simulink model "imsimulation"  (R2013a)
settings: Solver=ode45  StartTime=0.0  StopTime=10  RelTol=1e-3
values from neighbouring files (symbols this model uses):
  J = 0.089    [matlab.mat]
  P = 4    [matlab.mat]
  Rr = 0.816    [matlab.mat]
  Rs = 0.49    [matlab.mat]
  theta = 0    [matlab.mat]
  Wb = 157    [matlab.mat]
  We = 157    [matlab.mat]
  Xlr = 0.754    [matlab.mat]
  Xls = 0.754    [matlab.mat]
  Xm = 26.13    [matlab.mat]
undefined symbols (not defined in the file or in its folder): sigbuilder_block
settings Model: Creator=Administrator  LastModifiedBy=User
settings DebuggingCC: MultiTaskDSMMsg=warning  MultiTaskCondExecSysMsg=none  FcnCallInpInsideContextMsg=EnableAllAsWarning  StrictBusMsg=None
settings RTWCC: IncludeERTFirstTime=on

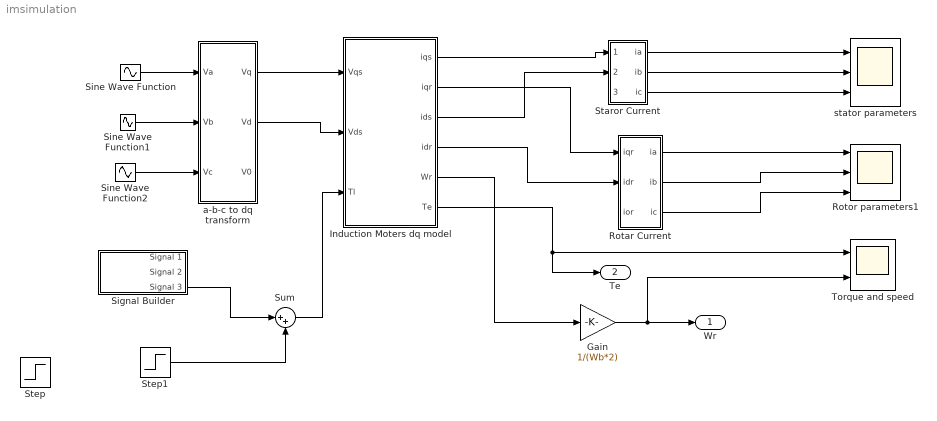
== system imsimulation ==
  Gain : Gain  Gain=1/(Wb*2)
  "Induction Moters dq model " : Subsystem
  Rotar Current : Subsystem
  Rotor parameters1 : Scope  NumInputPorts=3
      settings: YMin=-5~-5~-5  YMax=5~5~5
  Signal Builder : Subsystem  Tag=STV Subsys  LoadFcn=sigbuilder_block('load');  StartFcn=sigbuilder_block('start');  StopFcn=sigbuilder_block('stop');  ClipboardFcn=sigbuilder_block('clipboard');  mask(Sigbuilder block){}
      mask help: Simulink:masks:SigbuilderBlock_MD
      mask init:
      | if ~strcmp(get_param(bdroot(gcbh),'SimulationStatus'),'stopped') tuvar = sigbuilder_block('maskInit'); end
      settings: CopyFcn=sigbuilder_block('copy');  DeleteFcn=sigbuilder_block('delete');  ModelCloseFcn=sigbuilder_block('modelClose');  PreSaveFcn=sigbuilder_block('preSave');  PauseFcn=sigbuilder_block('pause');  ContinueFcn=sigbuilder_block('continue');  NameChangeFcn=sigbuilder_block('namechange');  OpenFcn=sigbuilder_block('open',[6 30.75 1012.5 481.5 ]);  CloseFcn=sigbuilder_block('close');
      mask Display: plot(0, 0, 100, 100,[2, 2, 32, 32, 2], [68, 8, 8, 68, 68],[32, 2], [38, 38], [32, 19, 2],[53, 60, 44], [32, 17, 17, 2],[16, 16, 31, 31]);txt = getActiveGroup(gcbh);text(2, 100, txt,'verticalAlignment', 'top');
  Sine Wave Function : Sin  Amplitude=311.11  Frequency=50*2*pi  SampleTime=0
  Sine Wave Function1 : Sin  Amplitude=311.11  Frequency=50*2*pi  Phase=0-(2*pi/3)  SampleTime=0
  Sine Wave Function2 : Sin  Amplitude=311.11  Frequency=50*2*pi  Phase=0+(2*pi/3)  SampleTime=0
  "Staror Current " : Subsystem
  Step : Step  Time=3  After=11.95  SampleTime=0
  Step1 : Step  Time=6  After=-11.9  SampleTime=0
  Sum : Sum  Inputs=|++
  "Torque and speed " : Scope  NumInputPorts=2
      settings: TimeRange=0.1239454679989271  YMin=-60~-0.2  YMax=100~1.6  SaveName=ScopeData2
  "a-b-c to dq transform " : Subsystem
  stator parameters : Scope  NumInputPorts=3
      settings: TimeRange=1  YMin=-100~-100~-100  YMax=100~100~100
  Wr : Outport
  Te : Outport  Port=2
  wires:
  Sine Wave Function/1 -> "a-b-c to dq transform "/1(Va)
  Sine Wave Function1/1 -> "a-b-c to dq transform "/2(Vb)
  Sine Wave Function2/1 -> "a-b-c to dq transform "/3(Vc)
  "a-b-c to dq transform "/1(Vq) -> "Induction Moters dq model "/1(Vqs)
  "a-b-c to dq transform "/2(Vd) -> "Induction Moters dq model "/2(Vds)
  "Induction Moters dq model "/1(iqs) -> "Staror Current "/1(iqs)
  "Induction Moters dq model "/3(ids) -> "Staror Current "/2(ids)
  "Induction Moters dq model "/4(idr) -> Rotar Current/2(idr)
  "Induction Moters dq model "/2(iqr) -> Rotar Current/1(iqr)
  "Staror Current "/1(ia) -> stator parameters/1
  Rotar Current/1(ia) -> Rotor parameters1/1
  Rotar Current/2(ib) -> Rotor parameters1/2
  "Induction Moters dq model "/6(Te) -> Te/1, "Torque and speed "/1
  Step1/1 -> Sum/2
  "Induction Moters dq model "/5(Wr) -> Gain/1
  Sum/1 -> "Induction Moters dq model "/3(Tl)
  Gain/1 -> "Torque and speed "/2, Wr/1
  "Staror Current "/2(ib) -> stator parameters/2
  "Staror Current "/3("ic ") -> stator parameters/3
  Rotar Current/3("ic ") -> Rotor parameters1/3
  Signal Builder/3(Signal 3) -> Sum/1

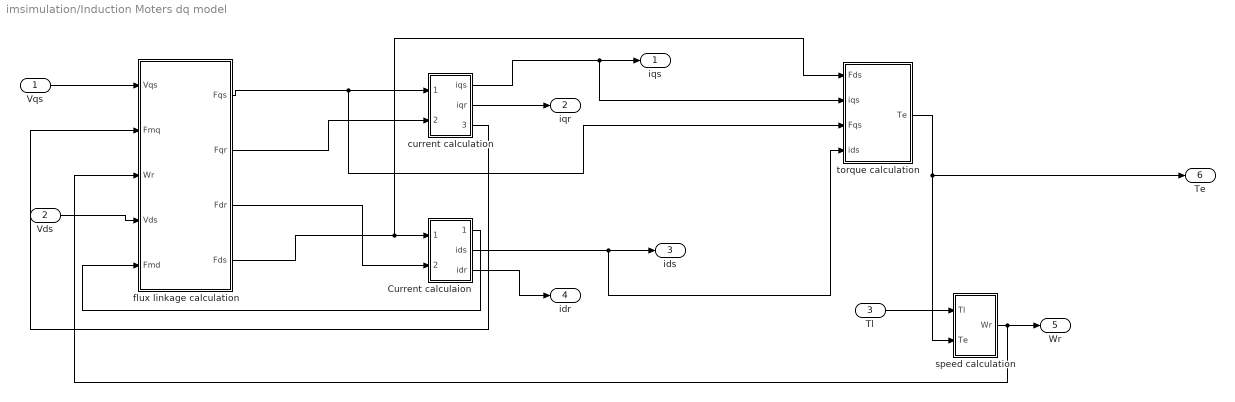
== system imsimulation/Induction Moters dq model  ==
  Vqs : Inport
  Vds : Inport  Port=2
  Tl : Inport  Port=3
  "Current calculaion " : Subsystem
  current calculation : Subsystem
  flux linkage calculation : Subsystem
  speed calculation : Subsystem
  "torque calculation " : Subsystem
  iqs : Outport
  iqr : Outport  Port=2
  ids : Outport  Port=3
  idr : Outport  Port=4
  Wr : Outport  Port=5
  Te : Outport  Port=6
  wires:
  Tl/1 -> speed calculation/1(Tl)
  "Current calculaion "/1(Fmd) -> flux linkage calculation/5(Fmd)
  current calculation/2(iqr) -> iqr/1
  current calculation/1(iqs) -> iqs/1, "torque calculation "/2(iqs)
  flux linkage calculation/3(Fdr) -> "Current calculaion "/2(Fdr)
  "Current calculaion "/2(ids) -> ids/1, "torque calculation "/4(ids)
  "Current calculaion "/3(idr) -> idr/1
  "torque calculation "/1(Te) -> Te/1, speed calculation/2(Te)
  flux linkage calculation/1(Fqs) -> "torque calculation "/3(Fqs), current calculation/1(Fqs)
  Vqs/1 -> flux linkage calculation/1(Vqs)
  Vds/1 -> flux linkage calculation/4(Vds)
  flux linkage calculation/2(Fqr) -> current calculation/2(Fqr)
  current calculation/3(Fmq) -> flux linkage calculation/2(Fmq)
  speed calculation/1(Wr) -> Wr/1, flux linkage calculation/3(Wr)
  flux linkage calculation/4(Fds) -> "torque calculation "/1(Fds), "Current calculaion "/1(Fds)

== system imsimulation/Rotar Current ==
  iqr : Inport
  idr : Inport  Port=2
  ior : Inport  Port=3
  Subsystem : Subsystem
  Subsystem1 : Subsystem
  Subsystem2 : Subsystem
  ia : Outport
  ib : Outport  Port=2
  "ic " : Outport  Port=3
  wires:
  Subsystem2/1("ic ") -> "ic "/1
  Subsystem1/1(ib) -> ib/1
  ior/1 -> Subsystem2/3(i0r), Subsystem/3(i0r), Subsystem1/3(i0r)
  idr/1 -> Subsystem2/2(idr), Subsystem/2(idr), Subsystem1/2(idr)
  iqr/1 -> Subsystem/1(iqr), Subsystem1/1(iqr), Subsystem2/1(iqr)
  Subsystem/1(ia) -> ia/1

== system imsimulation/Signal Builder ==
  Demux : Demux  Tag=STV Demux  Outputs=3
  FromWs : FromWorkspace  Tag=STV FromWs  VariableName=tuvar  SampleTime=0
      SigBuilderData=|
      | common.afterFinalStr = 'Extrapolate'
      | common.sampleTime = 0
      | dataSet.timeRange = [0 10]
      | dataSet.name = 'Group 1'
      | sbobj.Groups.Name = 'Group 1'
      | sbobj.Groups.Signals(1).Name = 'Signal 1'
      | sbobj.Groups.Signals(1).XData = [0 4 6 6 10]
      | sbobj.Groups.Signals(1).YData = [0 1.005 1 1.005 0.995]
      | sbobj.Groups.Signals(2).Name = 'Signal 2'
      | sbobj.Groups.Signals(2).XData = [0 0.5 0.5 1 1 1.5 1.5 2 2 2.5 2.5 3 3 3.5 3.5 4 4 4.5 4.5 5 5 5.5 5.5 6 6 6.5 6.5 7 7 7.5 7.5 8 8 8.5 8.5 9 9 9.5 9.5 10]
      | sbobj.Groups.Signals(2).YData = [2 2 0 0 2 2 0 0 2 2 0 0 2 2 0 0 2 2 0 0 2 2 0 0 2 2 0 0 2 2 0 0 2 2 0 0 2 2 0 0]
      | sbobj.Groups.Signals(3).Name = 'Signal 3'
      | sbobj.Groups.Signals(3).XData = [0 10]
      | sbobj.Groups.Signals(3).YData = [1 1]
  Signal 1 : Outport  Tag=STV Outport
  Signal 2 : Outport  Tag=STV Outport  Port=2
  Signal 3 : Outport  Tag=STV Outport  Port=3
  wires:
  Demux/1 -> Signal 1/1
  FromWs/1 -> Demux/1
  Demux/2 -> Signal 2/1
  Demux/3 -> Signal 3/1

== system imsimulation/Staror Current  ==
  iqs : Inport
  ids : Inport  Port=2
  ios : Inport  Port=3
  Subsystem : Subsystem
  Subsystem1 : Subsystem
  Subsystem2 : Subsystem
  ia : Outport
  ib : Outport  Port=2
  "ic " : Outport  Port=3
  wires:
  Subsystem/1(ia) -> ia/1
  iqs/1 -> Subsystem2/1(iqs), Subsystem1/1(iqs), Subsystem/1(iqs)
  ids/1 -> Subsystem1/2(ids), Subsystem/2(ids), Subsystem2/2(ids)
  ios/1 -> Subsystem1/3(i0s), Subsystem/3(i0s), Subsystem2/3(i0)
  Subsystem1/1(ib) -> ib/1
  Subsystem2/1("ic ") -> "ic "/1

== system imsimulation/a-b-c to dq transform  ==
  Va : Inport
  Vb : Inport  Port=2
  Vc : Inport  Port=3
  Subsystem : Subsystem
  Subsystem1 : Subsystem
  Subsystem2 : Subsystem
  Vq : Outport
  Vd : Outport  Port=2
  V0 : Outport  Port=3
  wires:
  Vc/1 -> Subsystem2/3(Vc), Subsystem1/3(Vc), Subsystem/3(Vc)
  Vb/1 -> Subsystem/2(Vb), Subsystem1/2(Vb), Subsystem2/2(Vb)
  Subsystem/1(Vq) -> Vq/1
  Subsystem1/1("Vd ") -> Vd/1
  Va/1 -> Subsystem1/1(Va), Subsystem/1(Va), Subsystem2/1(Va)
  Subsystem2/1(V0) -> V0/1

== system imsimulation/Induction Moters dq model /Current calculaion  ==
  Fds : Inport
  Fdr : Inport  Port=2
  Subsystem1 : Subsystem
  Subsystem4 : Subsystem
  Subsystem5 : Subsystem
  Fmd : Outport
  ids : Outport  Port=2
  idr : Outport  Port=3
  wires:
  Subsystem1/1(Fmd) -> Fmd/1, Subsystem4/2(Fmd), Subsystem5/2(Fmd)
  Fdr/1 -> Subsystem5/1(Fdr), Subsystem1/2(Fdr)
  Fds/1 -> Subsystem4/1(Fds), Subsystem1/1(Fds)
  Subsystem4/1(ids) -> ids/1
  Subsystem5/1(idr) -> idr/1

== system imsimulation/Induction Moters dq model /current calculation ==
  Fqs : Inport
  Fqr : Inport  Port=2
  Subsystem : Subsystem
  Subsystem2 : Subsystem
  Subsystem3 : Subsystem
  iqs : Outport
  iqr : Outport  Port=2
  Fmq : Outport  Port=3
  wires:
  Subsystem2/1(iqs) -> iqs/1
  Subsystem/1(Fmq) -> Fmq/1, Subsystem2/2(Fmq), Subsystem3/2(Fmq)
  Subsystem3/1(iqr) -> iqr/1
  Fqs/1 -> Subsystem/1(Fqs), Subsystem2/1(Fqs)
  Fqr/1 -> Subsystem/2(Fqr), Subsystem3/1(Fqr)

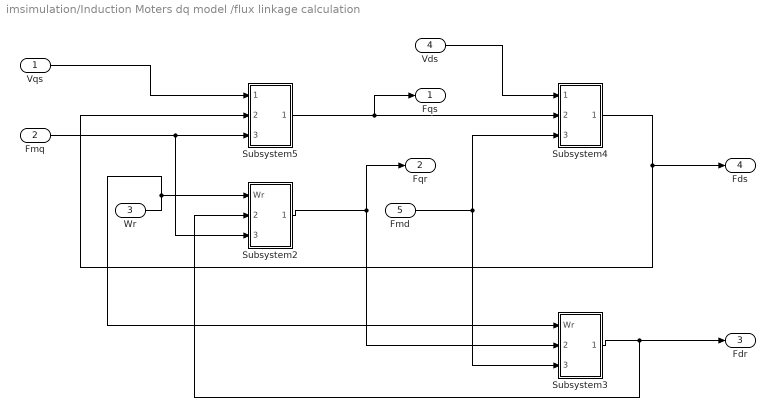
== system imsimulation/Induction Moters dq model /flux linkage calculation ==
  Vqs : Inport
  Fmq : Inport  Port=2
  Wr : Inport  Port=3
  Vds : Inport  Port=4
  Fmd : Inport  Port=5
  Subsystem2 : Subsystem
  Subsystem3 : Subsystem
  Subsystem4 : Subsystem
  Subsystem5 : Subsystem
  Fqs : Outport
  Fqr : Outport  Port=2
  Fdr : Outport  Port=3
  Fds : Outport  Port=4
  wires:
  Subsystem2/1(Fqr) -> Fqr/1, Subsystem3/2(Fqr)
  Wr/1 -> Subsystem3/1(Wr), Subsystem2/1(Wr)
  Vqs/1 -> Subsystem5/1(Vqs)
  Vds/1 -> Subsystem4/1(Vds)
  Fmq/1 -> Subsystem2/3(Fmq), Subsystem5/3(Fmq)
  Subsystem5/1(Fqs) -> Fqs/1, Subsystem4/2(Fqs)
  Subsystem4/1(Fds) -> Fds/1, Subsystem5/2(Fds)
  Subsystem3/1(Fdr) -> Fdr/1, Subsystem2/2(Fdr)
  Fmd/1 -> Subsystem3/3(Fmd), Subsystem4/3(Fmd)

== system imsimulation/Induction Moters dq model /speed calculation ==
  Tl : Inport
  Te : Inport  Port=2
  Add : Sum  Inputs=+-
  Gain : Gain  Gain=P/(2*J)
  Integrator : Integrator
  Wr : Outport
  wires:
  Add/1 -> Gain/1
  Tl/1 -> Add/2
  Te/1 -> Add/1
  Gain/1 -> Integrator/1
  Integrator/1 -> Wr/1

== system imsimulation/Induction Moters dq model /torque calculation  ==
  Fds : Inport
  iqs : Inport  Port=2
  Fqs : Inport  Port=3
  ids : Inport  Port=4
  Add : Sum  Inputs=+-
  Gain : Gain  Gain=1.5*P/(2*Wb)
  Product : Product
  Product1 : Product
  Te : Outport
  wires:
  Product/1 -> Add/1
  iqs/1 -> Product/2
  ids/1 -> Product1/2
  Fds/1 -> Product/1
  Fqs/1 -> Product1/1
  Product1/1 -> Add/2
  Gain/1 -> Te/1
  Add/1 -> Gain/1

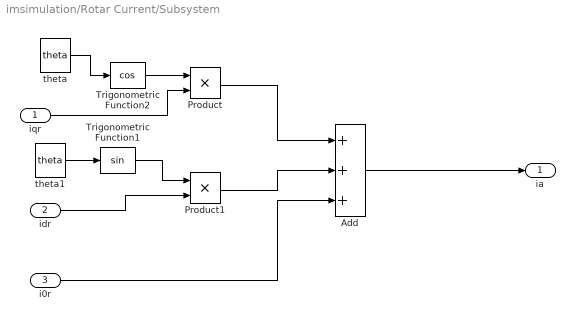
== system imsimulation/Rotar Current/Subsystem ==
  iqr : Inport
  idr : Inport  Port=2
  i0r : Inport  Port=3
  Add : Sum  Inputs=+++
  Product : Product
  Product1 : Product
  Trigonometric Function1 : Trigonometry
  Trigonometric Function2 : Trigonometry  Operator=cos
  theta : Constant  Value=theta  VectorParams1D=off
  theta1 : Constant  Value=theta  VectorParams1D=off
  ia : Outport
  wires:
  Add/1 -> ia/1
  i0r/1 -> Add/3
  idr/1 -> Product1/2
  Trigonometric Function1/1 -> Product1/1
  theta/1 -> Trigonometric Function2/1
  iqr/1 -> Product/2
  Trigonometric Function2/1 -> Product/1
  theta1/1 -> Trigonometric Function1/1
  Product1/1 -> Add/2
  Product/1 -> Add/1

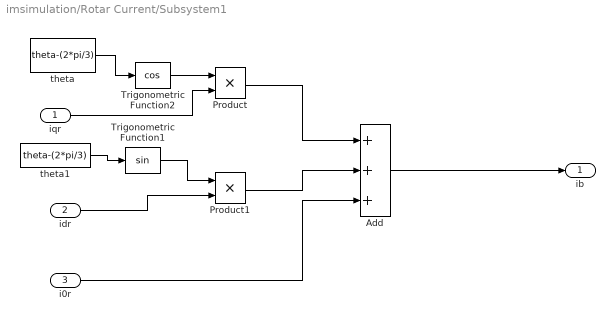
== system imsimulation/Rotar Current/Subsystem1 ==
  iqr : Inport
  idr : Inport  Port=2
  i0r : Inport  Port=3
  Add : Sum  Inputs=+++
  Product : Product
  Product1 : Product
  Trigonometric Function1 : Trigonometry
  Trigonometric Function2 : Trigonometry  Operator=cos
  theta : Constant  Value=theta-(2*pi/3)  VectorParams1D=off
  theta1 : Constant  Value=theta-(2*pi/3)  VectorParams1D=off
  ib : Outport
  wires:
  Product1/1 -> Add/2
  theta1/1 -> Trigonometric Function1/1
  Trigonometric Function2/1 -> Product/1
  iqr/1 -> Product/2
  theta/1 -> Trigonometric Function2/1
  Trigonometric Function1/1 -> Product1/1
  idr/1 -> Product1/2
  i0r/1 -> Add/3
  Add/1 -> ib/1
  Product/1 -> Add/1

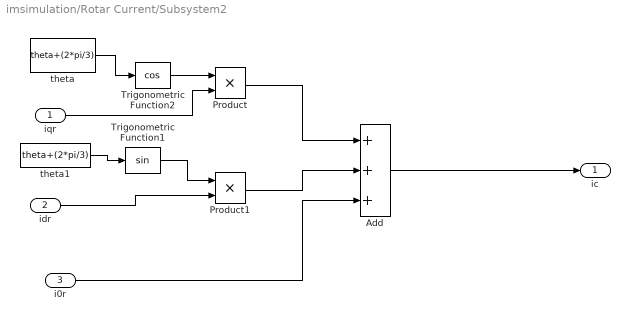
== system imsimulation/Rotar Current/Subsystem2 ==
  iqr : Inport
  idr : Inport  Port=2
  i0r : Inport  Port=3
  Add : Sum  Inputs=+++
  Product : Product
  Product1 : Product
  Trigonometric Function1 : Trigonometry
  Trigonometric Function2 : Trigonometry  Operator=cos
  theta : Constant  Value=theta+(2*pi/3)  VectorParams1D=off
  theta1 : Constant  Value=theta+(2*pi/3)  VectorParams1D=off
  "ic " : Outport
  wires:
  Product1/1 -> Add/2
  theta1/1 -> Trigonometric Function1/1
  Trigonometric Function2/1 -> Product/1
  iqr/1 -> Product/2
  theta/1 -> Trigonometric Function2/1
  Trigonometric Function1/1 -> Product1/1
  idr/1 -> Product1/2
  i0r/1 -> Add/3
  Add/1 -> "ic "/1
  Product/1 -> Add/1

== system imsimulation/Staror Current /Subsystem ==
  iqs : Inport
  ids : Inport  Port=2
  i0s : Inport  Port=3
  Add : Sum  Inputs=+++
  Product : Product
  Product1 : Product
  Trigonometric Function1 : Trigonometry
  Trigonometric Function2 : Trigonometry  Operator=cos
  theta : Constant  Value=theta  VectorParams1D=off
  theta1 : Constant  Value=theta  VectorParams1D=off
  ia : Outport
  wires:
  Product/1 -> Add/1
  Product1/1 -> Add/2
  theta1/1 -> Trigonometric Function1/1
  Trigonometric Function2/1 -> Product/1
  iqs/1 -> Product/2
  theta/1 -> Trigonometric Function2/1
  Trigonometric Function1/1 -> Product1/1
  ids/1 -> Product1/2
  i0s/1 -> Add/3
  Add/1 -> ia/1

== system imsimulation/Staror Current /Subsystem1 ==
  iqs : Inport
  ids : Inport  Port=2
  i0s : Inport  Port=3
  Add : Sum  Inputs=+++
  Product : Product
  Product1 : Product
  Trigonometric Function1 : Trigonometry
  Trigonometric Function2 : Trigonometry  Operator=cos
  theta : Constant  Value=theta-(2*pi/3)  VectorParams1D=off
  theta1 : Constant  Value=theta-(2*pi/3)  VectorParams1D=off
  ib : Outport
  wires:
  Product/1 -> Add/1
  Add/1 -> ib/1
  i0s/1 -> Add/3
  ids/1 -> Product1/2
  Trigonometric Function1/1 -> Product1/1
  theta/1 -> Trigonometric Function2/1
  iqs/1 -> Product/2
  Trigonometric Function2/1 -> Product/1
  theta1/1 -> Trigonometric Function1/1
  Product1/1 -> Add/2

== system imsimulation/Staror Current /Subsystem2 ==
  note: s
  iqs : Inport
  ids : Inport  Port=2
  i0 : Inport  Port=3
  Add : Sum  Inputs=+++
  Product : Product
  Product1 : Product
  Trigonometric Function1 : Trigonometry
  Trigonometric Function2 : Trigonometry  Operator=cos
  theta : Constant  Value=theta+(2*pi/3)  VectorParams1D=off
  theta1 : Constant  Value=theta+(2*pi/3)  VectorParams1D=off
  "ic " : Outport
  wires:
  Product/1 -> Add/1
  Add/1 -> "ic "/1
  i0/1 -> Add/3
  ids/1 -> Product1/2
  Trigonometric Function1/1 -> Product1/1
  theta/1 -> Trigonometric Function2/1
  iqs/1 -> Product/2
  Trigonometric Function2/1 -> Product/1
  theta1/1 -> Trigonometric Function1/1
  Product1/1 -> Add/2

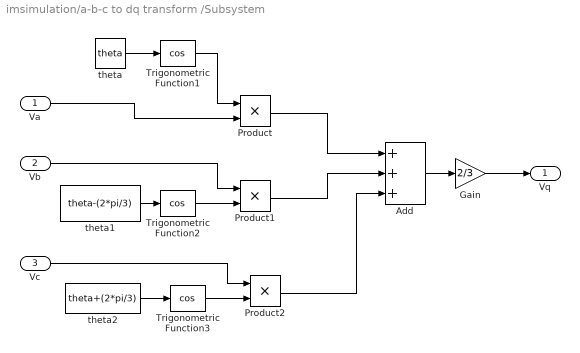
== system imsimulation/a-b-c to dq transform /Subsystem ==
  Va : Inport
  Vb : Inport  Port=2
  Vc : Inport  Port=3
  Add : Sum  Inputs=+++
  Gain : Gain  Gain=2/3
  Product : Product
  Product1 : Product
  Product2 : Product
  Trigonometric Function1 : Trigonometry  Operator=cos
  Trigonometric Function2 : Trigonometry  Operator=cos
  Trigonometric Function3 : Trigonometry  Operator=cos
  theta : Constant  Value=theta
  theta1 : Constant  Value=theta-(2*pi/3)
  theta2 : Constant  Value=theta+(2*pi/3)
  Vq : Outport
  wires:
  theta/1 -> Trigonometric Function1/1
  Vb/1 -> Product1/1
  Trigonometric Function2/1 -> Product1/2
  Vc/1 -> Product2/1
  Va/1 -> Product/2
  Trigonometric Function3/1 -> Product2/2
  theta1/1 -> Trigonometric Function2/1
  Trigonometric Function1/1 -> Product/1
  Add/1 -> Gain/1
  theta2/1 -> Trigonometric Function3/1
  Gain/1 -> Vq/1
  Product2/1 -> Add/3
  Product/1 -> Add/1
  Product1/1 -> Add/2

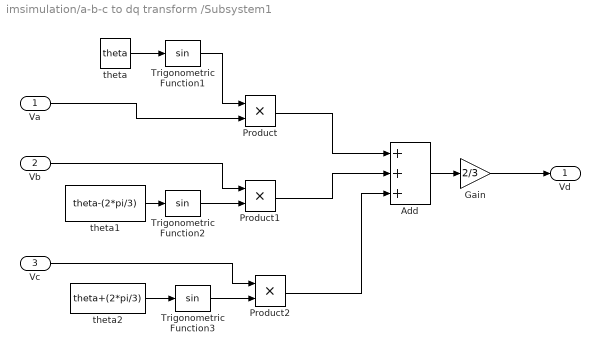
== system imsimulation/a-b-c to dq transform /Subsystem1 ==
  Va : Inport
  Vb : Inport  Port=2
  Vc : Inport  Port=3
  Add : Sum  Inputs=+++
  Gain : Gain  Gain=2/3
  Product : Product
  Product1 : Product
  Product2 : Product
  Trigonometric Function1 : Trigonometry
  Trigonometric Function2 : Trigonometry
  Trigonometric Function3 : Trigonometry
  theta : Constant  Value=theta
  theta1 : Constant  Value=theta-(2*pi/3)
  theta2 : Constant  Value=theta+(2*pi/3)
  "Vd " : Outport
  wires:
  Trigonometric Function3/1 -> Product2/2
  theta/1 -> Trigonometric Function1/1
  Trigonometric Function1/1 -> Product/1
  Vc/1 -> Product2/1
  Product2/1 -> Add/3
  theta2/1 -> Trigonometric Function3/1
  Trigonometric Function2/1 -> Product1/2
  Gain/1 -> "Vd "/1
  Product1/1 -> Add/2
  Vb/1 -> Product1/1
  Product/1 -> Add/1
  Add/1 -> Gain/1
  theta1/1 -> Trigonometric Function2/1
  Va/1 -> Product/2

== system imsimulation/a-b-c to dq transform /Subsystem2 ==
  Va : Inport
  Vb : Inport  Port=2
  Vc : Inport  Port=3
  Add : Sum  Inputs=+++
  Gain : Gain  Gain=1/3
  V0 : Outport
  wires:
  Gain/1 -> V0/1
  Va/1 -> Add/1
  Vb/1 -> Add/2
  Vc/1 -> Add/3
  Add/1 -> Gain/1

== system imsimulation/Induction Moters dq model /Current calculaion /Subsystem1 ==
  Fds : Inport
  Fdr : Inport  Port=2
  Add1 : Sum
  Gain3 : Gain  Gain=1/((1/Xm)+(1/Xls)+(1/Xlr))
  Gain4 : Gain  Gain=1/Xls
  Gain5 : Gain  Gain=1/Xlr
  Fmd : Outport
  wires:
  Gain5/1 -> Add1/2
  Gain3/1 -> Fmd/1
  Fds/1 -> Gain4/1
  Fdr/1 -> Gain5/1
  Add1/1 -> Gain3/1
  Gain4/1 -> Add1/1

== system imsimulation/Induction Moters dq model /Current calculaion /Subsystem4 ==
  Fds : Inport
  Fmd : Inport  Port=2
  Add2 : Sum  Inputs=+-
  Gain2 : Gain  Gain=1/Xls
  ids : Outport
  wires:
  Gain2/1 -> ids/1
  Add2/1 -> Gain2/1
  Fmd/1 -> Add2/2
  Fds/1 -> Add2/1

== system imsimulation/Induction Moters dq model /Current calculaion /Subsystem5 ==
  Fdr : Inport
  Fmd : Inport  Port=2
  Add3 : Sum  Inputs=-+
  Gain3 : Gain  Gain=1/Xlr
  idr : Outport
  wires:
  Add3/1 -> Gain3/1
  Fdr/1 -> Add3/2
  Gain3/1 -> idr/1
  Fmd/1 -> Add3/1

== system imsimulation/Induction Moters dq model /current calculation/Subsystem ==
  Fqs : Inport
  Fqr : Inport  Port=2
  Add : Sum
  Gain : Gain  Gain=1/((1/Xm)+(1/Xls)+(1/Xlr))
  Gain1 : Gain  Gain=1/Xls
  Gain2 : Gain  Gain=1/Xlr
  Fmq : Outport
  wires:
  Fqs/1 -> Gain1/1
  Gain2/1 -> Add/2
  Add/1 -> Gain/1
  Fqr/1 -> Gain2/1
  Gain1/1 -> Add/1
  Gain/1 -> Fmq/1

== system imsimulation/Induction Moters dq model /current calculation/Subsystem2 ==
  Fqs : Inport
  Fmq : Inport  Port=2
  Add : Sum  Inputs=+-
  Gain : Gain  Gain=1/Xls
  iqs : Outport
  wires:
  Fqs/1 -> Add/1
  Fmq/1 -> Add/2
  Gain/1 -> iqs/1
  Add/1 -> Gain/1

== system imsimulation/Induction Moters dq model /current calculation/Subsystem3 ==
  Fqr : Inport
  Fmq : Inport  Port=2
  Add1 : Sum  Inputs=-+
  Gain1 : Gain  Gain=1/Xlr
  iqr : Outport
  wires:
  Gain1/1 -> iqr/1
  Add1/1 -> Gain1/1
  Fqr/1 -> Add1/2
  Fmq/1 -> Add1/1

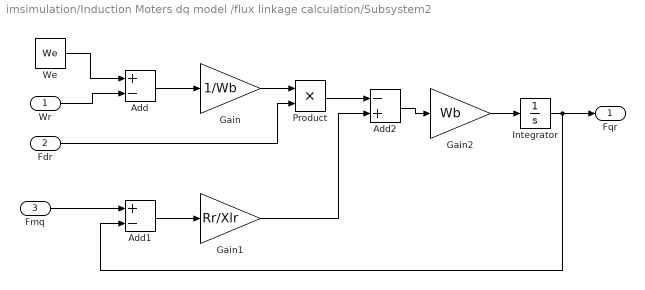
== system imsimulation/Induction Moters dq model /flux linkage calculation/Subsystem2 ==
  Wr : Inport
  Fdr : Inport  Port=2
  Fmq : Inport  Port=3
  Add : Sum  Inputs=+-
  Add1 : Sum  Inputs=+-
  Add2 : Sum  Inputs=-+
  Gain : Gain  Gain=1/Wb
  Gain1 : Gain  Gain=Rr/Xlr
  Gain2 : Gain  Gain=Wb
  Integrator : Integrator
  Product : Product
  We : Constant  Value=We
  Fqr : Outport
  wires:
  Fmq/1 -> Add1/1
  Fdr/1 -> Product/2
  Gain1/1 -> Add2/2
  Add/1 -> Gain/1
  Add1/1 -> Gain1/1
  Add2/1 -> Gain2/1
  Gain2/1 -> Integrator/1
  Product/1 -> Add2/1
  Gain/1 -> Product/1
  Wr/1 -> Add/2
  We/1 -> Add/1
  Integrator/1 -> Fqr/1, Add1/2

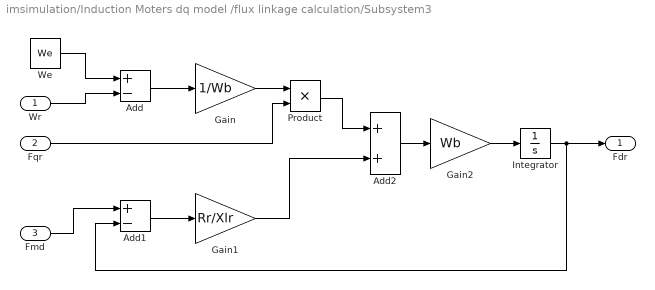
== system imsimulation/Induction Moters dq model /flux linkage calculation/Subsystem3 ==
  Wr : Inport
  Fqr : Inport  Port=2
  Fmd : Inport  Port=3
  Add : Sum  Inputs=+-
  Add1 : Sum  Inputs=+-
  Add2 : Sum
  Gain : Gain  Gain=1/Wb
  Gain1 : Gain  Gain=Rr/Xlr
  Gain2 : Gain  Gain=Wb
  Integrator : Integrator
  Product : Product
  We : Constant  Value=We
  Fdr : Outport
  wires:
  Add2/1 -> Gain2/1
  Integrator/1 -> Fdr/1, Add1/2
  Wr/1 -> Add/2
  Gain2/1 -> Integrator/1
  Gain/1 -> Product/1
  Fqr/1 -> Product/2
  We/1 -> Add/1
  Product/1 -> Add2/1
  Gain1/1 -> Add2/2
  Fmd/1 -> Add1/1
  Add1/1 -> Gain1/1
  Add/1 -> Gain/1

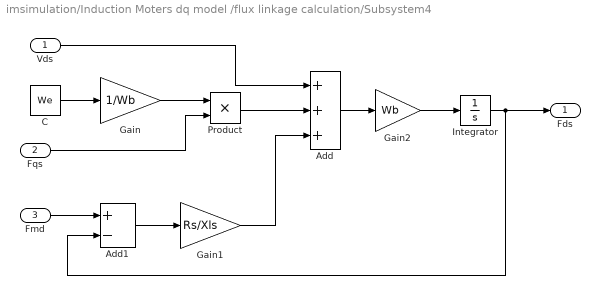
== system imsimulation/Induction Moters dq model /flux linkage calculation/Subsystem4 ==
  Vds : Inport
  Fqs : Inport  Port=2
  Fmd : Inport  Port=3
  Add : Sum  Inputs=+++
  Add1 : Sum  Inputs=+-
  C : Constant  Value=We
  Gain : Gain  Gain=1/Wb
  Gain1 : Gain  Gain=Rs/Xls
  Gain2 : Gain  Gain=Wb
  Integrator : Integrator
  Product : Product
  Fds : Outport
  wires:
  Integrator/1 -> Fds/1, Add1/2
  Gain2/1 -> Integrator/1
  Add1/1 -> Gain1/1
  Gain1/1 -> Add/3
  Vds/1 -> Add/1
  Product/1 -> Add/2
  Fqs/1 -> Product/2
  Add/1 -> Gain2/1
  C/1 -> Gain/1
  Fmd/1 -> Add1/1
  Gain/1 -> Product/1

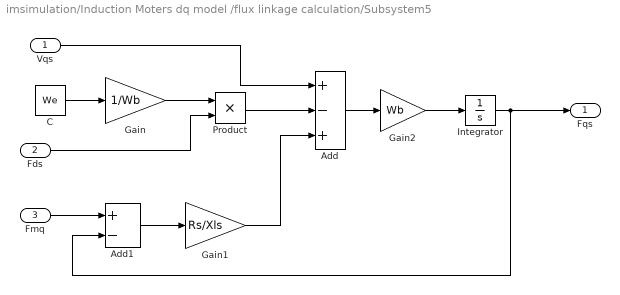
== system imsimulation/Induction Moters dq model /flux linkage calculation/Subsystem5 ==
  Vqs : Inport
  Fds : Inport  Port=2
  Fmq : Inport  Port=3
  Add : Sum  Inputs=+-+
  Add1 : Sum  Inputs=+-
  C : Constant  Value=We
  Gain : Gain  Gain=1/Wb
  Gain1 : Gain  Gain=Rs/Xls
  Gain2 : Gain  Gain=Wb
  Integrator : Integrator
  Product : Product
  Fqs : Outport
  wires:
  Vqs/1 -> Add/1
  Gain1/1 -> Add/3
  Fds/1 -> Product/2
  Product/1 -> Add/2
  Fmq/1 -> Add1/1
  Integrator/1 -> Fqs/1, Add1/2
  Add1/1 -> Gain1/1
  Gain2/1 -> Integrator/1
  Add/1 -> Gain2/1
  C/1 -> Gain/1
  Gain/1 -> Product/1
